simulink model "acc"  (R2021b)
settings: Solver=FixedStepAuto  StartTime=0.0  StopTime=inf  FixedStep=0.01  RelTol=1e-3
settings Model: DataDictionary=acc.sldd  EnableAccessToBaseWorkspace=off  Creator=pc  LastModifiedBy=pc

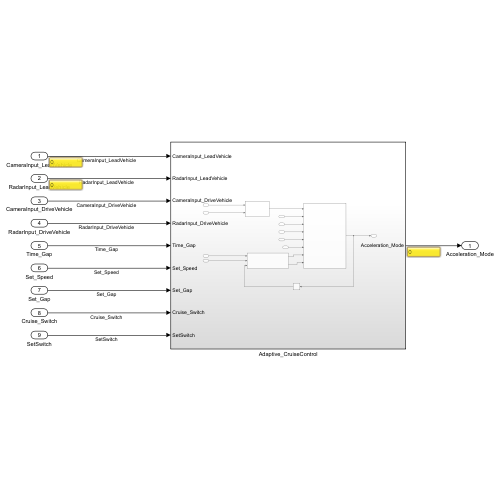
[thumbnail: Simulink's stored preview of the top-level diagram]
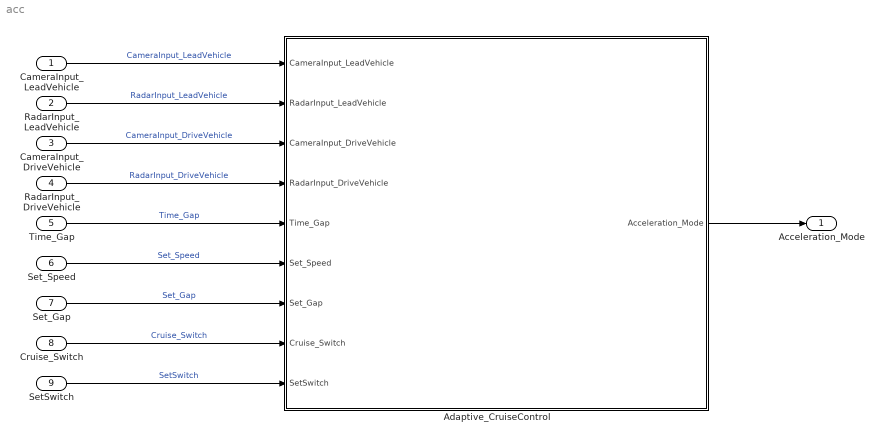
== system acc ==
  CameraInput_LeadVehicle : Inport  OutMin=0  OutMax=255  OutDataTypeStr=uint8
  RadarInput_LeadVehicle : Inport  Port=2  OutMin=0  OutMax=255  OutDataTypeStr=uint8
  CameraInput_DriveVehicle : Inport  Port=3  OutMin=0  OutMax=255  OutDataTypeStr=uint8
  RadarInput_DriveVehicle : Inport  Port=4  OutMin=0  OutMax=255  OutDataTypeStr=uint8
  Time_Gap : Inport  Port=5  OutMin=0  OutMax=255  OutDataTypeStr=uint8
  Set_Speed : Inport  Port=6  OutMin=0  OutMax=255  OutDataTypeStr=uint8
  Set_Gap : Inport  Port=7  OutMin=0  OutMax=255  OutDataTypeStr=uint8
  Cruise_Switch : Inport  Port=8  OutMin=0  OutMax=1  OutDataTypeStr=boolean
  SetSwitch : Inport  Port=9  OutMin=0  OutMax=1  OutDataTypeStr=boolean
  Adaptive_CruiseControl : Subsystem
  Acceleration_Mode : Outport  OutMin=0  OutMax=255  OutDataTypeStr=uint8
  wires:
  CameraInput_LeadVehicle/1 -> Adaptive_CruiseControl/1(CameraInput_LeadVehicle)  "CameraInput_LeadVehicle"
  RadarInput_LeadVehicle/1 -> Adaptive_CruiseControl/2(RadarInput_LeadVehicle)  "RadarInput_LeadVehicle"
  CameraInput_DriveVehicle/1 -> Adaptive_CruiseControl/3(CameraInput_DriveVehicle)  "CameraInput_DriveVehicle"
  RadarInput_DriveVehicle/1 -> Adaptive_CruiseControl/4(RadarInput_DriveVehicle)  "RadarInput_DriveVehicle"
  Time_Gap/1 -> Adaptive_CruiseControl/5(Time_Gap)  "Time_Gap"
  Set_Speed/1 -> Adaptive_CruiseControl/6(Set_Speed)  "Set_Speed"
  Set_Gap/1 -> Adaptive_CruiseControl/7(Set_Gap)  "Set_Gap"
  Cruise_Switch/1 -> Adaptive_CruiseControl/8(Cruise_Switch)  "Cruise_Switch"
  SetSwitch/1 -> Adaptive_CruiseControl/9(SetSwitch)  "SetSwitch"
  Adaptive_CruiseControl/1(Acceleration_Mode) -> Acceleration_Mode/1

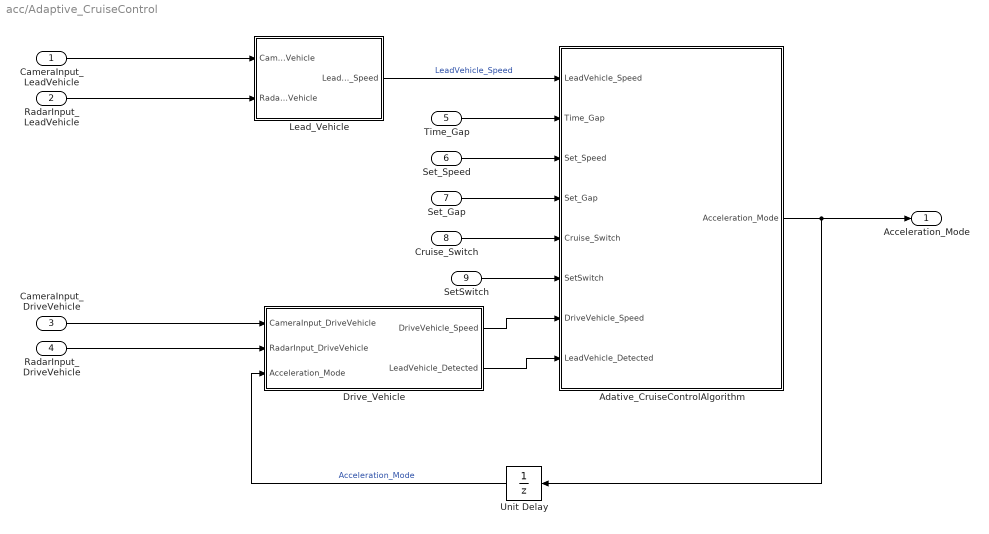
== system acc/Adaptive_CruiseControl ==
  CameraInput_LeadVehicle : Inport
  RadarInput_LeadVehicle : Inport  Port=2
  CameraInput_DriveVehicle : Inport  Port=3
  RadarInput_DriveVehicle : Inport  Port=4
  Time_Gap : Inport  Port=5
  Set_Speed : Inport  Port=6
  Set_Gap : Inport  Port=7
  Cruise_Switch : Inport  Port=8
  SetSwitch : Inport  Port=9
  Adative_CruiseControlAlgorithm : Subsystem
  Drive_Vehicle : Subsystem
  Lead_Vehicle : Subsystem
  Unit Delay : UnitDelay  SampleTime=-1  HasFrameUpgradeWarning=on
  Acceleration_Mode : Outport
  wires:
  CameraInput_LeadVehicle/1 -> Lead_Vehicle/1(CameraInput_LeadVehicle)
  RadarInput_LeadVehicle/1 -> Lead_Vehicle/2(RadarInput_LeadVehicle)
  CameraInput_DriveVehicle/1 -> Drive_Vehicle/1(CameraInput_DriveVehicle)
  RadarInput_DriveVehicle/1 -> Drive_Vehicle/2(RadarInput_DriveVehicle)
  Adative_CruiseControlAlgorithm/1(Acceleration_Mode) -> Unit Delay/1, Acceleration_Mode/1
  Unit Delay/1 -> Drive_Vehicle/3(Acceleration_Mode)  "Acceleration_Mode"
  Lead_Vehicle/1(LeadVehicle_Speed) -> Adative_CruiseControlAlgorithm/1(LeadVehicle_Speed)  "LeadVehicle_Speed"
  Time_Gap/1 -> Adative_CruiseControlAlgorithm/2(Time_Gap)
  Drive_Vehicle/1(DriveVehicle_Speed) -> Adative_CruiseControlAlgorithm/7(DriveVehicle_Speed)
  Drive_Vehicle/2(LeadVehicle_Detected) -> Adative_CruiseControlAlgorithm/8(LeadVehicle_Detected)
  SetSwitch/1 -> Adative_CruiseControlAlgorithm/6(SetSwitch)
  Cruise_Switch/1 -> Adative_CruiseControlAlgorithm/5(Cruise_Switch)
  Set_Gap/1 -> Adative_CruiseControlAlgorithm/4(Set_Gap)
  Set_Speed/1 -> Adative_CruiseControlAlgorithm/3(Set_Speed)

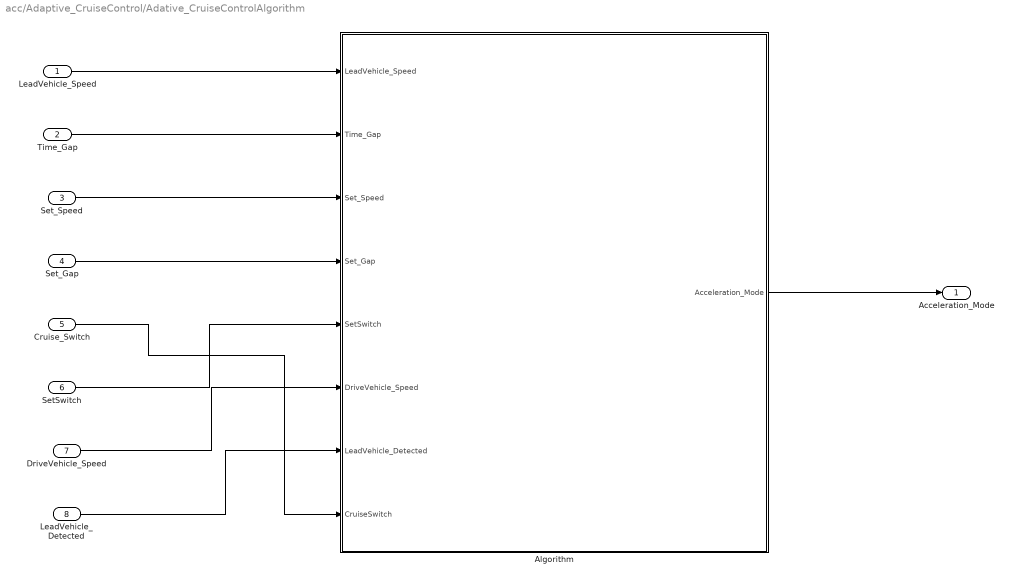
== system acc/Adaptive_CruiseControl/Adative_CruiseControlAlgorithm ==
  LeadVehicle_Speed : Inport
  Time_Gap : Inport  Port=2
  Set_Speed : Inport  Port=3
  Set_Gap : Inport  Port=4
  Cruise_Switch : Inport  Port=5
  SetSwitch : Inport  Port=6
  DriveVehicle_Speed : Inport  Port=7
  LeadVehicle_Detected : Inport  Port=8
  Algorithm : Stateflow chart  TreatAsAtomicUnit=on
  Acceleration_Mode : Outport  OutMin=0  OutMax=255  OutDataTypeStr=uint8
  wires:
  Algorithm/1(Acceleration_Mode) -> Acceleration_Mode/1
  LeadVehicle_Speed/1 -> Algorithm/1(LeadVehicle_Speed)
  Time_Gap/1 -> Algorithm/2(Time_Gap)
  Set_Speed/1 -> Algorithm/3(Set_Speed)
  Set_Gap/1 -> Algorithm/4(Set_Gap)
  SetSwitch/1 -> Algorithm/5(SetSwitch)
  DriveVehicle_Speed/1 -> Algorithm/6(DriveVehicle_Speed)
  LeadVehicle_Detected/1 -> Algorithm/7(LeadVehicle_Detected)
  Cruise_Switch/1 -> Algorithm/8(CruiseSwitch)

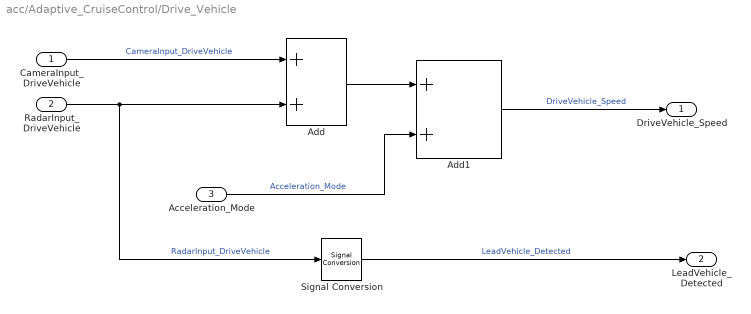
== system acc/Adaptive_CruiseControl/Drive_Vehicle ==
  CameraInput_DriveVehicle : Inport
  RadarInput_DriveVehicle : Inport  Port=2
  Acceleration_Mode : Inport  Port=3
  Add : Sum
  Add1 : Sum
  Signal Conversion : SignalConversion  OverrideOpt=off
  DriveVehicle_Speed : Outport
  LeadVehicle_Detected : Outport  Port=2
  wires:
  CameraInput_DriveVehicle/1 -> Add/1  "CameraInput_DriveVehicle"
  RadarInput_DriveVehicle/1 -> Signal Conversion/1, Add/2  "RadarInput_DriveVehicle"
  Add/1 -> Add1/1
  Acceleration_Mode/1 -> Add1/2  "Acceleration_Mode"
  Add1/1 -> DriveVehicle_Speed/1  "DriveVehicle_Speed"
  Signal Conversion/1 -> LeadVehicle_Detected/1  "LeadVehicle_Detected"

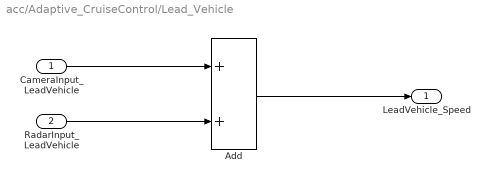
== system acc/Adaptive_CruiseControl/Lead_Vehicle ==
  CameraInput_LeadVehicle : Inport
  RadarInput_LeadVehicle : Inport  Port=2
  Add : Sum
  LeadVehicle_Speed : Outport
  wires:
  Add/1 -> LeadVehicle_Speed/1
  CameraInput_LeadVehicle/1 -> Add/1
  RadarInput_LeadVehicle/1 -> Add/2

== stateflow chart acc/Adaptive_CruiseControl/Adative_CruiseControlAlgorithm/Algorithm ==
  state ACC_OFF_MODE
    entry:
    Acceleration_Mode == 0;
  state ACC_STANDBY_MODE
    entry:
    Acceleration_Mode == 1;
  state ACC_ON_MODE
    state LeadVehicle_Detected_Follow
      entry:
      Acceleration_Mode == 2;
    state LeadVehicle_Detected_Resume
      entry:
      Acceleration_Mode == 3;
    state LeadVehicle_Not_Detected_Resume
      entry:
      Acceleration_Mode == 1;
    state LeadVehicle_Not_Detected
      entry:
      Acceleration_Mode == 1;
    state LeadVehicle_Speed_lessthan_Set_Speed
      entry:
      Acceleration_Mode == 4;
    state LeadVehicle_Speed_equal_Set_Speed
      entry:
      Acceleration_Mode == 5;
    (default) -> LeadVehicle_Detected_Follow
    LeadVehicle_Detected_Resume -> LeadVehicle_Detected_Follow [order 1] : [(DriveVehicle_Speed == Set_Speed) &&...
        | (LeadVehicle_Speed >= Set_Speed) &&...
        | (Time_Gap >= Set_Gap)]
    LeadVehicle_Detected_Resume -> LeadVehicle_Not_Detected_Resume [order 3] : [LeadVehicle_Detected == 0]
    LeadVehicle_Detected_Follow -> LeadVehicle_Not_Detected : [LeadVehicle_Detected == 0]
    LeadVehicle_Not_Detected -> LeadVehicle_Detected_Follow [order 1] : [(LeadVehicle_Detected == 1) &&...
        | (DriveVehicle_Speed == Set_Speed) &&...
        | (LeadVehicle_Speed >= Set_Speed) &&...
        | (Time_Gap >= Set_Gap)]
    LeadVehicle_Speed_equal_Set_Speed -> LeadVehicle_Not_Detected_Resume [order 3] : [(LeadVehicle_Detected==0)||...
        | (DriveVehicle_Speed<=Set_Speed)]
    LeadVehicle_Detected_Resume -> LeadVehicle_Speed_equal_Set_Speed [order 2] : [(DriveVehicle_Speed < Set_Speed) &&...
        | (LeadVehicle_Speed > DriveVehicle_Speed) &&...
        | (Time_Gap >= Set_Gap)]
    LeadVehicle_Speed_equal_Set_Speed -> LeadVehicle_Detected_Resume [order 2] : [(DriveVehicle_Speed < Set_Speed) &&...
        | (LeadVehicle_Speed > DriveVehicle_Speed)||...
        | (Time_Gap >= Set_Gap)]
    LeadVehicle_Not_Detected -> LeadVehicle_Speed_lessthan_Set_Speed [order 2] : [(LeadVehicle_Detected == 1) &&...
        | (LeadVehicle_Speed < Set_Speed)||...
        | (Time_Gap < Set_Gap)]
    LeadVehicle_Speed_lessthan_Set_Speed -> LeadVehicle_Not_Detected [order 1] : [(LeadVehicle_Detected == 0) &&...
        | (DriveVehicle_Speed == Set_Speed)]
    LeadVehicle_Speed_lessthan_Set_Speed -> LeadVehicle_Speed_equal_Set_Speed [order 2] : [((LeadVehicle_Speed*1.25 >= DriveVehicle_Speed) &&...
        | (LeadVehicle_Speed*0.75 <= DriveVehicle_Speed)) &&...
        | (DriveVehicle_Speed < Set_Speed) &&...
        | ((Time_Gap <= 1.25*Set_Gap) &&...
        | (Time_Gap <= 0.75*Set_Gap))]
    LeadVehicle_Speed_equal_Set_Speed -> LeadVehicle_Speed_lessthan_Set_Speed [order 1] : [(LeadVehicle_Speed < Set_Speed) &&...
        | (LeadVehicle_Speed < DriveVehicle_Speed)||...
        | (Time_Gap == 0.75*Set_Gap)]
  (default) -> ACC_OFF_MODE
  ACC_OFF_MODE -> ACC_STANDBY_MODE : [CruiseSwitch == 1]
  ACC_STANDBY_MODE -> ACC_OFF_MODE [order 1] : [CruiseSwitch == 0]
  ACC_STANDBY_MODE -> ACC_ON_MODE [order 2] : [SetSwitch == 1]
  ACC_ON_MODE -> ACC_STANDBY_MODE : [SetSwitch == 0]
  data: Acceleration_Mode output; LeadVehicle_Speed input; Time_Gap input; Set_Speed input; Set_Gap input; SetSwitch input; DriveVehicle_Speed input; LeadVehicle_Detected input; CruiseSwitch input
